simulink model "roll_loop"  (R2014b)
settings: Solver=ode45  StartTime=0.0  StopTime=10.0  MaxStep=0.1  RelTol=1e-3
values from neighbouring files (symbols this model uses):
  a_phi_1 = -(1/2)*P.rho * Va^2 * P.S_wing * P.b * P.C_p_p * P.b / (2*Va)    [tuning.m]
  a_phi_2 = (1/2)*P.rho * Va^2 * P.S_wing * P.b * P.C_p_delta_a    [tuning.m]
  k_d_phi = (2*zeta_phi*w_n_phi - a_phi_1)/a_phi_2    [tuning.m]
  k_i_phi = 0.25    [tuning.m]
  k_p_phi = delta_a_max/e_phi_max * sign(a_phi_2)    [tuning.m]
settings Model: Creator=kunalmenda  LastModifiedBy=kunalmenda

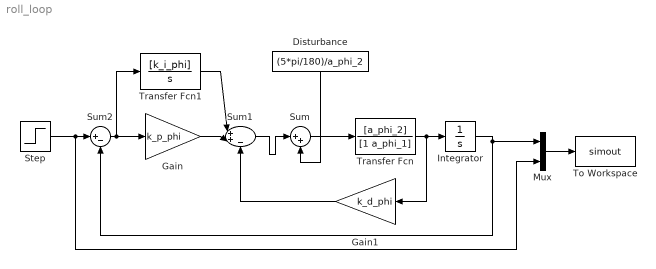
== system roll_loop ==
  Disturbance : Constant  Value=(5*pi/180)/a_phi_2
  Gain : Gain  Gain=k_p_phi
  Gain1 : Gain  Gain=k_d_phi
  Integrator : Integrator
  Mux : Mux  Inputs=2
  Step : Step  After=10*pi/180  SampleTime=0
  Sum : Sum  Inputs=|++
  Sum1 : Sum  Inputs=|++-
  Sum2 : Sum  Inputs=|+-
  To Workspace : ToWorkspace  VariableName=simout  SaveFormat=Timeseries  SampleTime=-1
  Transfer Fcn : TransferFcn  Numerator=[a_phi_2]  Denominator=[1 a_phi_1]
  Transfer Fcn1 : TransferFcn  Numerator=[k_i_phi]  Denominator=[1 0]
  wires:
  Sum2/1 -> Transfer Fcn1/1, Gain/1
  Transfer Fcn/1 -> Gain1/1, Integrator/1
  Sum/1 -> Transfer Fcn/1
  Sum1/1 -> Sum/1
  Disturbance/1 -> Sum/2
  Integrator/1 -> Mux/1, Sum2/2
  Step/1 -> Mux/2, Sum2/1
  Gain1/1 -> Sum1/3
  Gain/1 -> Sum1/2
  Transfer Fcn1/1 -> Sum1/1
  Mux/1 -> To Workspace/1
